simulink model "formation_planner_exp_cs"  (R2022b)
settings: Solver=ode5  StartTime=0.0  StopTime=80  FixedStep=1/1000  RelTol=1e-3
PreLoadFcn:
  | mbxruntime.callbacks.PreLoadFcn(bdroot);
PostLoadFcn:
  | mbxruntime.callbacks.PostLoadFcn(bdroot);
InitFcn:
  | mbxruntime.callbacks.InitFcn(bdroot);
StartFcn:
  | mbxruntime.callbacks.StartFcn(bdroot);
StopFcn:
  | mbxruntime.callbacks.StopFcn(bdroot);
model workspace (MAT data in the model file):
  mbox_table : object (value not decoded)
  model_closed = 0
  sim_status = 0
values from neighbouring files (symbols this model uses):
  c_factor = 43.75    [emplanner_init.m]
  car1_s = -10    [emplanner_init.m]
  car2_s = -20    [emplanner_init.m]
  cf = -175016    [emplanner_init.m]
  cr = -130634    [emplanner_init.m]
  KD_PID_distance = 0.0    (= 0)    [emplanner_init.m]
  KD_PID_speed = 0    [emplanner_init.m]
  KI_PID_distance = 0.0    (= 0)    [emplanner_init.m]
  KI_PID_speed = 0    [emplanner_init.m]
  KP_PID_distance = 0.5    [emplanner_init.m]
  KP_PID_speed = 1.8    [emplanner_init.m]
  la = 1.265    [emplanner_init.m]
  lb = 2.947-1.265    (= 1.682)    [emplanner_init.m]
  leader_global_kappa = global_kappa    [kappa.m]    (also in leader_global_path.mat = [0 0 0 0 0 0 0 0 0 0 0 0 ... (801 elements, 801x1)])
  leader_global_path_x = x_orgin.Data    [kappa.m]    (also in leader_global_path.mat = [2.22044604925e-16 0.999382255067 1.99750536558 2.9943522493)
  leader_global_path_y = y.Data    [kappa.m]    (also in leader_global_path.mat = [2 2 2 2 2 2 2 2 2 2 2 2 ... (801 elements, 801x1)])
  leader_global_yaw = yaw.Data    [kappa.m]    (also in leader_global_path.mat = [0 0 0 0 0 0 0 0 0 0 0 0 ... (801 elements, 801x1)])
  LQR_K1 = k(:,1)'    [emplanner_init.m]
  LQR_K2 = k(:,2)'    [emplanner_init.m]
  LQR_K3 = k(:,3)'    [emplanner_init.m]
  LQR_K4 = k(:,4)'    [emplanner_init.m]
  m = 2020    [emplanner_init.m]
  rack_displacement = [-39.14 , -37.2 , -35.29 , -33.43 , -31.6 , -29.81 , -28.06 , -26.34 , -24.66 ,      -23.01 , -21.38 , -19.79 , -18.23 , -16.69 , -15.18 , -13.7 , -12.23 , -10.8 , -9.38 , -7.98 ,     -6.61 , -5.25 , -3.91 , -2.59 , -1.29 , 0 , 1.27 , 2.54 , 3.78 , 5.02 , 6.24 , 7.46 , 8.66 ,      9.86 , 11.05 , 12.24 , 13.41 , 14.59 , 15.76 , 16.92 , 18.09 , 19.25 , 20.42 , 21.59 , 22.76 ,      23.93 , 25.11 , 26 ...(+26 chars)    [emplanner_init.m]
  right_wheel_ground = [-70 ,-67.2 , -64.4 , -61.6 , -58.8 , -56 , -53.2 , -50.4 , -47.6 , -44.8 , -42 ,      -39.2 , -36.4 , -33.6 , -30.8 , -28 , -25.2 , -22.4 , -19.6 , -16.8 , -14 , -11.2 , -8.4 , -5.6 ,      -2.8 , 0 , 2.8 , 5.6 , 8.4 , 11.2 , 14 , 16.8 , 19.6 , 22.4 , 25.2 , 28 , 30.8 , 33.6 , 36.4 ,      39.2 , 42 , 44.8 , 47.6 , 50.4 , 53.2 , 56 , 58.8 , 61.6 , 64.4 , 67.2 , 70 ]    [emplanner_init.m]
  vx_break_point = zeros(1,5000)    [emplanner_init.m]
undefined symbols (not defined in the file or in its folder): aubr, car1_global_kappa, car1_global_path_x, car1_global_path_y, car1_global_yaw, car2_global_kappa, car2_global_path_x, car2_global_path_y, car2_global_yaw, DiscIntNeverNeededParam, tablebr, vubr, warningInitialVelocity, x0
libraries: PreScanSimulinkLibrary x65, simulink x19, simulink_extras x14, Solver_SF x2
(part 12 of 31)

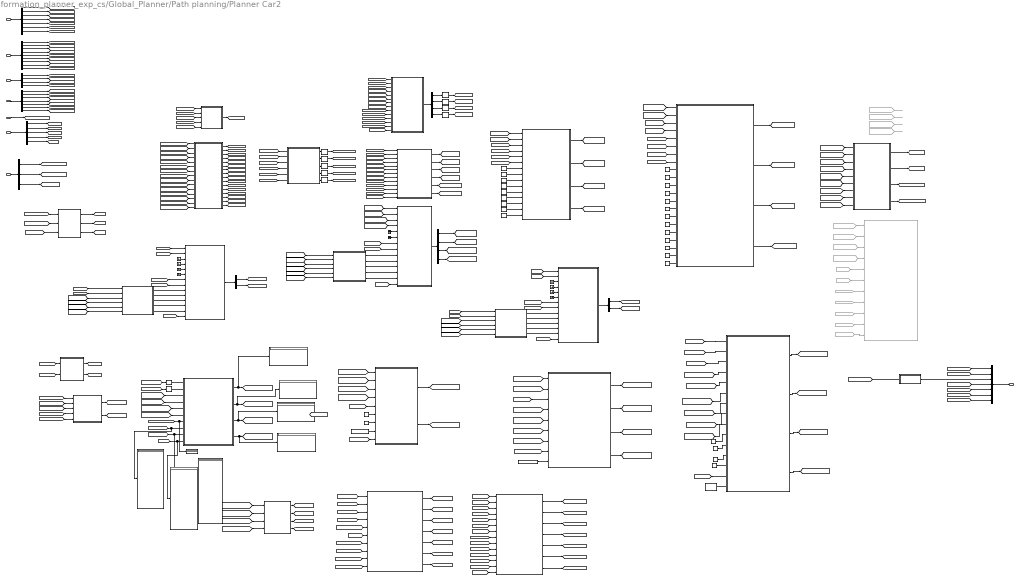
== system formation_planner_exp_cs/Global_Planner/Path planning/Planner Car2 ==
  referenceline info : Inport
  location info : Inport  Port=2
  perception info : Inport  Port=3
  pre_planning info : Inport  Port=4
  current time : Inport  Port=5
  leader_location_info : Inport  Port=6
  pre_car_result : Inport  Port=7
  Bus Creator : BusCreator  Inputs=7
  Bus Selector : BusSelector  OutputSignals=referenceline_x,referenceline_y,referenceline_heading,referenceline_kappa,origin_match_point_index,origin_x,origin_y
  Bus Selector1 : BusSelector  OutputSignals=host_x,host_y,host_heading_xy,host_vx,host_vy,host_yawrate,host_speed,host_ax,host_ay
  Bus Selector2 : BusSelector  OutputSignals=obs_x_set_gcs,obs_y_set_gcs,obs_velocity_set_gcs,obs_heading_set_gcs
  Bus Selector3 : BusSelector  OutputSignals=trajectory_x_gcs,trajectory_y_gcs,trajectory_heading_gcs,trajectory_kappa_gcs,trajectory_speed_gcs,trajectory_accel_gcs,trajectory_time_gcs
  Bus Selector4 : BusSelector  OutputSignals=s_set,l_set,dl_set,ddl_set
  Bus Selector5 : BusSelector  OutputSignals=s_set,l_set,s_dot_set,l_dot_set
  Bus Selector6 : BusSelector  OutputSignals=leader_x,leader_y,end_leader_x,end_leader_y,detla_t
  Bus Selector7 : BusSelector  OutputSignals=s_set,l_set
  Bus Selector8 : BusSelector  OutputSignals=trajectory_x_gcs,trajectory_y_gcs,trajectory_time_gcs
  Bus Selector9 : BusSelector  OutputSignals=s_set,l_set
  Cartesian2Frenet : Subsystem
  Cartesian2Frenet1 : Subsystem
  Cartesian2Frenet2 : Subsystem
  Cartesian2Frenet3 : Subsystem
  Constant : Constant  Value=1e6
  Constant1 : Constant  Value=2000
  Constant10 : Constant  Value=0.1
  Constant11 : Constant  Value=0.02
  Constant12 : Constant  Value=5
  Constant13 : Constant  Value=25000
  Constant14 : Constant  Value=50
  Constant15 : Constant  Value=20
  Constant{7,16..19} (5 alike) : Constant  Value=15
  Constant2 : Constant  Value=2
  Constant20 : Constant  Value=3
  Constant21 : Constant  Value=3
  Constant22 : Constant  Value=1.63
  Constant23 : Constant  Value=10
  Constant24 : Constant  Value=400
  Constant25 : Constant  Value=100
  Constant26 : Constant  Value=1000000000
  Constant27 : Constant  Value=0.2*9.8
  Constant28 : Constant  Value=50
  Constant29 : Constant  Value=500
  Constant3 : Constant  Value=3
  Constant30 : Constant  Value=20
  Constant34 : Constant  Value=car2_s
  Constant4 : Constant  Value=10
  Constant5 : Constant  Value=11
  Constant6 : Constant  Value=4
  Constant8 : Constant
  Constant9 : Constant  Value=10
  Delay : Delay  DelayLength=1
  Delay1 : Delay  DelayLength=1
  Display{,1..7} (8 alike) : Display
  Frenet2Cartesian task : MATLAB Function  TreatAsAtomicUnit=on
  From103 : From  Commented=on  GotoTag=dp_path_s_final
  From109 : From  Commented=on  GotoTag=dp_path_l_final
  From116 : From  Commented=on  GotoTag=dp_path_dl_final
  From117 : From  Commented=on  GotoTag=dp_path_ddl_final
  From120 : From  Commented=on  GotoTag=dp_path_s_final
  From124 : From  Commented=on  GotoTag=dp_path_l_final
  From125 : From  Commented=on  GotoTag=l_min
  From126 : From  Commented=on  GotoTag=l_max
  From129 : From  Commented=on  GotoTag=plan_start_l
  From130 : From  Commented=on  GotoTag=plan_start_dl
  From131 : From  Commented=on  GotoTag=plan_start_s
  From132 : From  Commented=on  GotoTag=static_obs_s_set
  From133 : From  Commented=on  GotoTag=static_obs_l_set
  From91 : From  Commented=on  GotoTag=qp_path_s_final
  From92 : From  Commented=on  GotoTag=qp_path_l_final
  Ground{,1..9} (10 alike) : Ground
  MATLAB Function : MATLAB Function  TreatAsAtomicUnit=on
  MATLAB Function1 : MATLAB Function  TreatAsAtomicUnit=on
  MATLAB Function2 : MATLAB Function  TreatAsAtomicUnit=on
  MATLAB Function3 : MATLAB Function  TreatAsAtomicUnit=on
  MATLAB Function4 : MATLAB Function  TreatAsAtomicUnit=on
  MATLAB Function5 : MATLAB Function  TreatAsAtomicUnit=on
  Selector{1..9} (9 alike) : Selector  InputPortWidth=128  IndexOptions=Index vector (dialog)  Indices=1  OutputSizes=1
  calc path length and map between point and s1 : MATLAB Function  TreatAsAtomicUnit=on
  calc plan start info and stitch trajectory : MATLAB Function  TreatAsAtomicUnit=on
  calc speed planning start condition : MATLAB Function  TreatAsAtomicUnit=on
  generate convex space : MATLAB Function  TreatAsAtomicUnit=on
  generate st graph : MATLAB Function  TreatAsAtomicUnit=on
  genrate index to s : MATLAB Function  TreatAsAtomicUnit=on
  increase st point count : MATLAB Function  TreatAsAtomicUnit=on
  obs : Subsystem
  path and speed merge : MATLAB Function  TreatAsAtomicUnit=on
  path decision task : Subsystem
  path planning task : Subsystem
  plot : MATLAB Function  Commented=on  TreatAsAtomicUnit=on
  speed decision with dynamic planning(dp) : MATLAB Function  TreatAsAtomicUnit=on
  speed planning with quadratic programming (qp) : MATLAB Function  TreatAsAtomicUnit=on
  stitch trajectory : MATLAB Function  TreatAsAtomicUnit=on
  EM Planner result : Outport
  wires:
  Constant30/1 -> speed planning with quadratic programming (qp)/13(w_cost_follow)
  [leader_poj_s] -> speed planning with quadratic programming (qp)/1(leader_poj_s)
  [trajectory_heading_init] -> MATLAB Function3/5(frenet_path_heading)
  MATLAB Function3/3(proj_y_set) -> Cartesian2Frenet2/11(proj_y_set)
  [trajectory_x_init] -> MATLAB Function3/3(frenet_path_x)
  MATLAB Function3/1(match_point_index_set) -> Cartesian2Frenet2/9(proj_match_point_index_set)
  MATLAB Function3/2(proj_x_set) -> Cartesian2Frenet2/10(proj_x_set)
  [trajectory_kappa_init] -> MATLAB Function3/6(frenet_path_kappa)
  [trajectory_x_init] -> Cartesian2Frenet2/7(frenet_path_x)
  [trajectory_y_init] -> Cartesian2Frenet2/8(frenet_path_y)
  [leader_start_x] -> MATLAB Function3/1(x_set)
  [leader_start_y] -> MATLAB Function3/2(y_set)
  MATLAB Function3/4(proj_heading_set) -> Cartesian2Frenet2/12(proj_heading_set)
  MATLAB Function3/5(proj_kappa_set) -> Cartesian2Frenet2/13(proj_kappa_set)
  [trajectory_y_init] -> MATLAB Function3/4(frenet_path_y)
  Bus Selector7/1 -> [leader_poj_s]  "<s_set>"
  [leader_start_x] -> Cartesian2Frenet2/1(x_set)
  Ground3/1 -> Cartesian2Frenet2/4(vy_set)
  Ground4/1 -> Cartesian2Frenet2/5(ax_set)
  Cartesian2Frenet2/1(Cartesian2FrenetOut) -> Bus Selector7/1
  Bus Selector7/2 -> [leader_poj_l]  "<l_set>"
  Ground5/1 -> Cartesian2Frenet2/6(ay_set)
  [leader_start_y] -> Cartesian2Frenet2/2(y_set)
  [path_index2s] -> Cartesian2Frenet2/14(index2s)
  Ground2/1 -> Cartesian2Frenet2/3(vx_set)
  Bus Selector6/5 -> [detla_t]  "<detla_t>"
  Bus Selector6/4 -> [leader_end_y]  "<end_leader_y>"
  Bus Selector6/3 -> [leader_end_x]  "<end_leader_x>"
  Bus Selector6/2 -> [leader_start_y]  "<leader_y>"
  Bus Selector6/1 -> [leader_start_x]  "<leader_x>"
  leader_location_info/1 -> Bus Selector6/1
  [host_speed] -> obs/4(host_speed)
  From109/1 -> ?
  From116/1 -> ?
  From117/1 -> ?
  From103/1 -> ?
  [qp_path_dl_final] -> Frenet2Cartesian task/3(dl_set)
  [qp_path_s_final] -> Frenet2Cartesian task/1(s_set)
  [qp_path_l_final] -> Frenet2Cartesian task/2(l_set)
  [qp_path_ddl_final] -> Frenet2Cartesian task/4(ddl_set)
  stitch trajectory/6(trajectory_accel_final) -> [trajectory_accel_final]
  [s_dot_lb] -> speed planning with quadratic programming (qp)/8(s_dot_lb)
  generate convex space/3(s_dot_lb) -> [s_dot_lb]
  generate st graph/1(obs_st_s_in_set) -> Display/1, [obs_st_s_in_set]
  [s] -> Delay/1
  [dp_speed_s] -> speed planning with quadratic programming (qp)/4(dp_speed_s)
  Constant29/1 -> speed planning with quadratic programming (qp)/12(w_cost_jerk)
  [stitch_y_gcs] -> stitch trajectory/9(stitch_y)
  Constant25/1 -> speed decision with dynamic planning(dp)/7(w_cost_accel)
  speed decision with dynamic planning(dp)/1(dp_speed_s) -> [dp_speed_s]
  [obs_st_t_out_set] -> speed decision with dynamic planning(dp)/4(obs_st_t_out_set)
  Constant23/1 -> [reference_speed]
  [dp_speed_t] -> speed planning with quadratic programming (qp)/5(dp_speed_t)
  [trajectory_heading] -> stitch trajectory/3(trajectory_heading)
  [plan_start_ay_gcs] -> calc speed planning start condition/4(plan_start_ay)
  [relative_time_init] -> increase st point count/4(relative_time_init)
  path and speed merge/1(trajectory_x) -> [trajectory_x]
  [trajectory_accel] -> stitch trajectory/6(trajectory_accel)
  [plan_start_ax_gcs] -> calc speed planning start condition/3(plan_start_ax)
  [stitch_speed_gcs] -> stitch trajectory/12(stitch_speed)
  [trajectory_speed] -> stitch trajectory/5(trajectory_speed)
  stitch trajectory/4(trajectory_kappa_final) -> [trajectory_kappa_final]
  speed planning with quadratic programming (qp)/4(relative_time_init) -> [relative_time_init]
  speed planning with quadratic programming (qp)/2(qp_s_dot_init) -> [qp_s_dot_init]
  [reference_speed] -> speed decision with dynamic planning(dp)/5(reference_speed_unlimit)
  [plan_start_s_dot] -> speed planning with quadratic programming (qp)/2(plan_start_s_dot)
  stitch trajectory/1(trajectory_x_final) -> [trajectory_x_final]
  [stitch_heading_gcs] -> stitch trajectory/10(stitch_heading)
  [stitch_accel_gcs] -> stitch trajectory/13(stitch_accel)
  [stitch_kappa_gcs] -> stitch trajectory/11(stitch_kappa)
  [stitch_time] -> stitch trajectory/14(stitch_time)
  [qp_s_init] -> increase st point count/1(s_init)
  [obs_st_s_in_set] -> speed decision with dynamic planning(dp)/1(obs_st_s_in_set)
  generate convex space/4(s_dot_ub) -> [s_dot_ub]
  [trajectory_y] -> stitch trajectory/2(trajectory_y)
  path and speed merge/2(trajectory_y) -> [trajectory_y]
  generate convex space/1(s_lb) -> [s_lb]
  [trajectory_kappa_init] -> path and speed merge/10(trajectory_kappa_init)
  path and speed merge/3(trajectory_heading) -> [trajectory_heading]
  [plan_start_s_dot2] -> speed planning with quadratic programming (qp)/3(plan_start_s_dot2)
  [trajectory_kappa] -> stitch trajectory/4(trajectory_kappa)
  [obs_st_s_in_set] -> generate convex space/4(obs_st_s_in_set)
  [trajectory_time] -> stitch trajectory/7(trajectory_time)
  [plan_start_time] -> path and speed merge/5(current_time)
  [s_ub] -> speed planning with quadratic programming (qp)/7(s_ub)
  [trajectory_y_init] -> path and speed merge/8(trajectory_y_init)
  [s_lb] -> speed planning with quadratic programming (qp)/6(s_lb)
  [trajectory_heading_init] -> path and speed merge/9(trajectory_heading_init)
  [path_index2s] -> path and speed merge/6(path_s)
  [qp_s_dot2_init] -> increase st point count/3(s_dot2_init)
  path and speed merge/5(trajectory_speed) -> [trajectory_speed]
  path and speed merge/7(trajectory_time) -> [trajectory_time]
  Constant26/1 -> speed decision with dynamic planning(dp)/8(w_cost_obs)
  [plan_start_heading_gcs] -> calc speed planning start condition/5(plan_start_heading)
  [obs_st_s_out_set] -> speed decision with dynamic planning(dp)/2(obs_st_s_out_set)
  Constant27/1 -> generate convex space/9(max_lateral_accel)
  [stitch_x_gcs] -> stitch trajectory/8(stitch_x)
  generate st graph/2(obs_st_s_out_set) -> Display1/1, [obs_st_s_out_set]
  speed decision with dynamic planning(dp)/2(dp_speed_t) -> [dp_speed_t]
  Constant9/1 -> speed planning with quadratic programming (qp)/10(w_cost_s_dot2)
  generate st graph/3(obs_st_t_in_set) -> Display2/1, [obs_st_t_in_set]
  speed planning with quadratic programming (qp)/1(qp_s_init) -> [qp_s_init]
  [relative_time] -> Delay1/1
  stitch trajectory/2(trajectory_y_final) -> [trajectory_y_final]
  [dynamic_obs_l_dot_set] -> generate st graph/6(dynamic_obs_l_dot_set)
  [s_dot_ub] -> speed planning with quadratic programming (qp)/9(s_dot_ub)
  [obs_st_t_in_set] -> speed decision with dynamic planning(dp)/3(obs_st_t_in_set)
  Constant28/1 -> speed planning with quadratic programming (qp)/11(w_cost_v_ref)
  calc speed planning start condition/1(plan_start_s_dot) -> [plan_start_s_dot]
  [reference_speed] -> speed planning with quadratic programming (qp)/14(speed_reference)
  speed planning with quadratic programming (qp)/3(qp_s_dot2_init) -> [qp_s_dot2_init]
  path and speed merge/4(trajectory_kappa) -> [trajectory_kappa]
  [dynamic_obs_s_dot_set] -> generate st graph/5(dynamic_obs_s_dot_set)
  [qp_s_dot_init] -> increase st point count/2(s_dot_init)
  [plan_start_s_dot] -> speed decision with dynamic planning(dp)/9(plan_start_s_dot)
  generate convex space/2(s_ub) -> [s_ub]
  [trajectory_kappa_init] -> generate convex space/8(trajectory_kappa_init)
  [obs_st_s_out_set] -> generate convex space/5(obs_st_s_out_set)
  [obs_st_t_out_set] -> generate convex space/7(obs_st_t_out_set)
  [obs_st_t_in_set] -> generate convex space/6(obs_st_t_in_set)
  [plan_start_vx_gcs] -> calc speed planning start condition/1(plan_start_vx)
  stitch trajectory/3(trajectory_heading_final) -> [trajectory_heading_final]
  [plan_start_vy_gcs] -> calc speed planning start condition/2(plan_start_vy)
  [s] -> path and speed merge/1(s)
  increase st point count/1(s) -> [s]
  [s_dot] -> path and speed merge/2(s_dot)
  [s_dot2] -> path and speed merge/3(s_dot2)
  [trajectory_x_init] -> path and speed merge/7(trajectory_x_init)
  calc speed planning start condition/2(plan_start_s_dot2) -> [plan_start_s_dot2]
  [relative_time] -> path and speed merge/4(relative_time)
  [trajectory_x] -> stitch trajectory/1(trajectory_x)
  path and speed merge/6(trajectory_accel) -> [trajectory_accel]
  Constant24/1 -> speed decision with dynamic planning(dp)/6(w_cost_ref_speed)
  generate st graph/4(obs_st_t_out_set) -> Display3/1, [obs_st_t_out_set]
  Delay1/1 -> generate st graph/2(pre_trajectory_t)
  stitch trajectory/7(trajectory_time_final) -> [trajectory_time_final]
  Delay/1 -> generate st graph/1(pre_trajectory_s)
  [dynamic_obs_s_set] -> generate st graph/3(dynamic_obs_s_set)
  increase st point count/3(s_dot2) -> [s_dot2]
  [path_index2s] -> generate convex space/3(path_index2s)
  stitch trajectory/5(trajectory_speed_final) -> [trajectory_speed_final]
  increase st point count/2(s_dot) -> [s_dot]
  [dynamic_obs_l_set] -> generate st graph/4(dynamic_obs_l_set)
  [dp_speed_s] -> generate convex space/1(dp_speed_s)
  increase st point count/4(relative_time) -> [relative_time]
  [dp_speed_t] -> generate convex space/2(dp_speed_t)
  Bus Selector5/4 -> [dynamic_obs_l_dot_set]  "<l_dot_set>"
  [dynamic_obs_x_set] -> Cartesian2Frenet1/1(x_set)
  Bus Selector5/3 -> [dynamic_obs_s_dot_set]  "<s_dot_set>"
  [trajectory_heading_init] -> MATLAB Function1/5(frenet_path_heading)
  [dynamic_obs_y_set] -> MATLAB Function1/2(y_set)
  [trajectory_y_init] -> Cartesian2Frenet1/8(frenet_path_y)
  Bus Selector5/2 -> [dynamic_obs_l_set]  "<l_set>"
  MATLAB Function1/1(match_point_index_set) -> Cartesian2Frenet1/9(proj_match_point_index_set)
  [trajectory_kappa_init] -> MATLAB Function1/6(frenet_path_kappa)
  Ground/1 -> Cartesian2Frenet1/5(ax_set)
  [path_index2s] -> Cartesian2Frenet1/14(index2s)
  [trajectory_x_init] -> Cartesian2Frenet1/7(frenet_path_x)
  Cartesian2Frenet1/1(Cartesian2FrenetOut) -> Bus Selector5/1
  MATLAB Function1/3(proj_y_set) -> Cartesian2Frenet1/11(proj_y_set)
  [dynamic_obs_vy_set] -> Cartesian2Frenet1/4(vy_set)
  [dynamic_obs_y_set] -> Cartesian2Frenet1/2(y_set)
  [dynamic_obs_vx_set] -> Cartesian2Frenet1/3(vx_set)
  [trajectory_y_init] -> MATLAB Function1/4(frenet_path_y)
  MATLAB Function1/2(proj_x_set) -> Cartesian2Frenet1/10(proj_x_set)
  MATLAB Function1/4(proj_heading_set) -> Cartesian2Frenet1/12(proj_heading_set)
  Ground1/1 -> Cartesian2Frenet1/6(ay_set)
  [dynamic_obs_x_set] -> MATLAB Function1/1(x_set)
  MATLAB Function1/5(proj_kappa_set) -> Cartesian2Frenet1/13(proj_kappa_set)
  [trajectory_x_init] -> MATLAB Function1/3(frenet_path_x)
  Bus Selector5/1 -> [dynamic_obs_s_set]  "<s_set>"
  calc path length and map between point and s1/1(path_s_end) -> [path_s_end]
  [trajectory_y_init] -> calc path length and map between point and s1/2(trajectory_y)
  calc path length and map between point and s1/2(path_index2s) -> [path_index2s]
  [trajectory_x_init] -> calc path length and map between point and s1/1(trajectory_x)
  [obs_x_set_gcs] -> obs/5(obs_x_set_gcs)
  obs/1(static_obs_s_set) -> [static_obs_s_set]
  [obs_y_set_gcs] -> obs/6(obs_y_set_gcs)
  [host_x] -> obs/1(host_x)
  [host_y] -> obs/2(host_y)
  [referenceline_kappa] -> obs/12(referenceline_kappa)
  [referenceline_heading] -> obs/11(referenceline_heading)
  [referenceline_x] -> obs/9(referenceline_x)
  [obs_heading_set_gcs] -> obs/8(obs_heading_set_gcs)
  [host_heading_xy] -> obs/3(host_heading_xy)
  [referenceline_y] -> obs/10(referenceline_y)
  [index2s] -> obs/13(index2s)
  obs/2(static_obs_l_set) -> [static_obs_l_set]
  obs/4(dynamic_obs_y_set) -> [dynamic_obs_y_set]
  obs/5(dynamic_obs_vx_set) -> [dynamic_obs_vx_set]
  obs/3(dynamic_obs_x_set) -> [dynamic_obs_x_set]
  obs/6(dynamic_obs_vy_set) -> [dynamic_obs_vy_set]
  [obs_velocity_set_gcs] -> obs/7(obs_velocity_set_gcs)
  MATLAB Function/1(y) -> Bus Creator/3  "trajectory_heading_gcs"
  [plan_start_s] -> path planning task/5(plan_start_s)
  From92/1 -> plot/4(qp_l)
  From91/1 -> plot/3(qp_s)
  path planning task/4(qp_path_ddl_final) -> [qp_path_ddl_final]
  path planning task/3(qp_path_dl_final) -> [qp_path_dl_final]
  path planning task/2(qp_path_l_final) -> [qp_path_l_final]
  path planning task/1(qp_path_s_final) -> [qp_path_s_final]
  Constant11/1 -> path planning task/21(delta_ddl_max)
  Constant10/1 -> path planning task/20(delta_dl_max)
  [static_obs_l_set] -> path planning task/4(static_obs_l_set)
  [static_obs_s_set] -> path planning task/3(static_obs_s_set)
  Constant2/1 -> path decision task/9(dp_cost_ddl)
  Constant1/1 -> path decision task/8(dp_cost_dl)
  Constant/1 -> path decision task/7(dp_cost_collision)
  Constant3/1 -> path decision task/10(dp_cost_dddl)
  Constant4/1 -> path decision task/11(dp_cost_ref)
  Constant5/1 -> path decision task/12(dp_row)
  Constant6/1 -> path decision task/13(dp_col)
  Constant7/1 -> path decision task/14(dp_sample_s)
  Constant8/1 -> path decision task/15(dp_sample_l)
  Constant12/1 -> path planning task/9(qp_cost_l)
  Constant13/1 -> path planning task/10(qp_cost_dl)
  Constant14/1 -> path planning task/11(qp_cost_ddl)
  Constant15/1 -> path planning task/12(qp_cost_dddl)
  Constant16/1 -> path planning task/13(qp_cost_centre)
  Constant17/1 -> path planning task/14(qp_cost_endl)
  Constant18/1 -> path planning task/15(qp_cost_end_dl)
  Constant19/1 -> path planning task/16(qp_cost_end_ddl)
  Constant20/1 -> path planning task/17(host_d1)
  Constant21/1 -> path planning task/18(host_d2)
  Constant22/1 -> path planning task/19(host_w)
  [plan_start_dl] -> path planning task/7(plan_start_dl)
  [plan_start_ddl] -> path planning task/8(plan_start_ddl)
  [plan_start_l] -> path planning task/6(plan_start_l)
  [dp_path_l_final] -> path planning task/2(dp_path_l_final)
  [dp_path_s_final] -> path planning task/1(dp_path_s_final)
  [plan_start_s] -> path decision task/3(plan_start_s)
  [plan_start_l] -> path decision task/4(plan_start_l)
  [plan_start_dl] -> path decision task/5(plan_start_dl)
  [plan_start_ddl] -> path decision task/6(plan_start_ddl)
  [static_obs_l_set] -> path decision task/2(static_obs_l_set)
  [static_obs_s_set] -> path decision task/1(static_obs_s_set)
  path decision task/4(dp_path_ddl_final) -> [dp_path_ddl_final]
  path decision task/3(dp_path_dl_final) -> [dp_path_dl_final]
  path decision task/2(dp_path_l_final) -> [dp_path_l_final]
  path decision task/1(dp_path_s_final) -> [dp_path_s_final]
  From133/1 -> plot/8(obs_l_set)
  From132/1 -> plot/7(obs_s_set)
  From131/1 -> plot/9(start_s)
  From129/1 -> plot/10(start_l)
  From130/1 -> plot/11(start_dl)
  From126/1 -> plot/6(l_max)
  From125/1 -> plot/5(l_min)
  From124/1 -> plot/2(dp_l)
  From120/1 -> plot/1(dp_s)
  Frenet2Cartesian task/4(kappa_set) -> [trajectory_kappa_init]
  Frenet2Cartesian task/3(heading_set) -> [trajectory_heading_init]
  Frenet2Cartesian task/2(y_set) -> [trajectory_y_init]
  Frenet2Cartesian task/1(x_set) -> [trajectory_x_init]
  [referenceline_kappa] -> Frenet2Cartesian task/8(frenet_path_kappa)
  [referenceline_heading] -> Frenet2Cartesian task/7(frenet_path_heading)
  [referenceline_y] -> Frenet2Cartesian task/6(frenet_path_y)
  [referenceline_x] -> Frenet2Cartesian task/5(frenet_path_x)
  [index2s] -> Frenet2Cartesian task/9(index2s)
  [trajectory_y_final] -> Bus Creator/2  "trajectory_y_gcs"
  [trajectory_kappa_final] -> Bus Creator/4  "trajectory_kappa_gcs"
  [trajectory_heading_final] -> MATLAB Function/1(trajectory_heading_final)
  [trajectory_speed_final] -> Bus Creator/5  "trajectory_speed_gcs"
  [trajectory_accel_final] -> Bus Creator/6  "trajectory_accel_gcs"
  [trajectory_time_final] -> Bus Creator/7  "trajectory_time_gcs"
  [trajectory_x_final] -> Bus Creator/1  "trajectory_x_gcs"
  Bus Creator/1 -> EM Planner result/1
  [index2s] -> Cartesian2Frenet/14(index2s)
  Selector9/1 -> [plan_start_ddl]
  Selector8/1 -> [plan_start_dl]
  Selector7/1 -> [plan_start_l]
  Selector6/1 -> [plan_start_s]
  Bus Selector4/1 -> Selector6/1  "<s_set>"
  Bus Selector4/2 -> Selector7/1  "<l_set>"
  Bus Selector4/3 -> Selector8/1  "<dl_set>"
  Bus Selector4/4 -> Selector9/1  "<ddl_set>"
  Cartesian2Frenet/1(Cartesian2FrenetOut) -> Bus Selector4/1
  [plan_start_proj_kappa] -> Cartesian2Frenet/13(proj_kappa_set)
  [plan_start_proj_heading] -> Cartesian2Frenet/12(proj_heading_set)
  [plan_start_proj_y] -> Cartesian2Frenet/11(proj_y_set)
  [plan_start_proj_x] -> Cartesian2Frenet/10(proj_x_set)
  [plan_start_match_point_index] -> Cartesian2Frenet/9(proj_match_point_index_set)
  [referenceline_y] -> Cartesian2Frenet/8(frenet_path_y)
  [referenceline_x] -> Cartesian2Frenet/7(frenet_path_x)
  [plan_start_ay_gcs] -> Cartesian2Frenet/6(ay_set)
  [plan_start_ax_gcs] -> Cartesian2Frenet/5(ax_set)
  [plan_start_vy_gcs] -> Cartesian2Frenet/4(vy_set)
  [plan_start_vx_gcs] -> Cartesian2Frenet/3(vx_set)
  [plan_start_x_gcs] -> Cartesian2Frenet/1(x_set)
  [plan_start_y_gcs] -> Cartesian2Frenet/2(y_set)
  Selector5/1 -> [plan_start_proj_kappa]
  Selector4/1 -> [plan_start_proj_heading]
  Selector3/1 -> [plan_start_proj_y]
  Selector2/1 -> [plan_start_proj_x]
  Selector1/1 -> [plan_start_match_point_index]
  [referenceline_kappa] -> MATLAB Function2/6(frenet_path_kappa)
  [referenceline_heading] -> MATLAB Function2/5(frenet_path_heading)
  [referenceline_y] -> MATLAB Function2/4(frenet_path_y)
  [referenceline_x] -> MATLAB Function2/3(frenet_path_x)
  [plan_start_y_gcs] -> MATLAB Function2/2(y_set)
  [plan_start_x_gcs] -> MATLAB Function2/1(x_set)
  MATLAB Function2/2(proj_x_set) -> Selector2/1
  MATLAB Function2/4(proj_heading_set) -> Selector4/1
  MATLAB Function2/1(match_point_index_set) -> Selector1/1
  MATLAB Function2/3(proj_y_set) -> Selector3/1
  MATLAB Function2/5(proj_kappa_set) -> Selector5/1
  genrate index to s/1(index2s) -> [index2s]
  [origin_match_point_index] -> genrate index to s/5(origin_match_point_index)
  [origin_y] -> genrate index to s/4(origin_y)
  [origin_x] -> genrate index to s/3(origin_x)
  [referenceline_y] -> genrate index to s/2(path_y)
  [referenceline_x] -> genrate index to s/1(path_x)
  Bus Selector/7 -> [origin_y]  "<origin_y>"
  Bus Selector/6 -> [origin_x]  "<origin_x>"
  Bus Selector/5 -> [origin_match_point_index]  "<origin_match_point_index>"
  calc plan start info and stitch trajectory/16(stitch_time) -> [stitch_time]
  calc plan start info and stitch trajectory/15(stitch_accel) -> [stitch_accel_gcs]
  calc plan start info and stitch trajectory/14(stitch_speed) -> [stitch_speed_gcs]
  calc plan start info and stitch trajectory/13(stitch_kappa) -> [stitch_kappa_gcs]
  calc plan start info and stitch trajectory/12(stitch_heading) -> [stitch_heading_gcs]
  calc plan start info and stitch trajectory/11(stitch_y) -> [stitch_y_gcs]
  calc plan start info and stitch trajectory/10(stitch_x) -> [stitch_x_gcs]
  calc plan start info and stitch trajectory/9(plan_start_time) -> [plan_start_time]
  calc plan start info and stitch trajectory/8(plan_start_ay) -> [plan_start_ay_gcs]
  calc plan start info and stitch trajectory/7(plan_start_ax) -> [plan_start_ax_gcs]
  calc plan start info and stitch trajectory/6(plan_start_vy) -> [plan_start_vy_gcs]
  calc plan start info and stitch trajectory/5(plan_start_vx) -> [plan_start_vx_gcs]
  calc plan start info and stitch trajectory/4(plan_start_kappa) -> [plan_start_kappa_gcs]
  calc plan start info and stitch trajectory/3(plan_start_heading) -> [plan_start_heading_gcs]
  calc plan start info and stitch trajectory/2(plan_start_y) -> [plan_start_y_gcs]
  calc plan start info and stitch trajectory/1(plan_start_x) -> [plan_start_x_gcs]
  [pre_trajectory_heading_gcs] -> calc plan start info and stitch trajectory/3(pre_trajectory_heading)
  [pre_trajectory_kappa_gcs] -> calc plan start info and stitch trajectory/4(pre_trajectory_kappa)
  [pre_trajectory_speed_gcs] -> calc plan start info and stitch trajectory/5(pre_trajectory_velocity)
  [pre_trajectory_accel_gcs] -> calc plan start info and stitch trajectory/6(pre_trajectory_accel)
  [pre_trajectory_time] -> calc plan start info and stitch trajectory/7(pre_trajectory_time)
  [pre_trajectory_y_gcs] -> calc plan start info and stitch trajectory/2(pre_trajectory_y)
  [pre_trajectory_x_gcs] -> calc plan start info and stitch trajectory/1(pre_trajectory_x)
  [current_time] -> calc plan start info and stitch trajectory/8(current_time)
  [host_x] -> calc plan start info and stitch trajectory/9(host_x)
  [host_y] -> calc plan start info and stitch trajectory/10(host_y)
  [host_heading_xy] -> calc plan start info and stitch trajectory/11(host_heading_xy)
  [host_vx_vcs] -> calc plan start info and stitch trajectory/12(host_vx)
  [host_vy_vcs] -> calc plan start info and stitch trajectory/13(host_vy)
  [host_ax_vcs] -> calc plan start info and stitch trajectory/14(host_ax)
  [host_ay_vcs] -> calc plan start info and stitch trajectory/15(host_ay)
  Bus Selector/4 -> [referenceline_kappa]  "<referenceline_kappa>"
  Bus Selector/3 -> [referenceline_heading]  "<referenceline_heading>"
  Bus Selector/2 -> [referenceline_y]  "<referenceline_y>"
  Bus Selector/1 -> [referenceline_x]  "<referenceline_x>"
  Bus Selector1/9 -> [host_ay_vcs]  "<host_ay>"
  Bus Selector1/8 -> [host_ax_vcs]  "<host_ax>"
  Bus Selector1/7 -> [host_speed]  "<host_speed>"
  Bus Selector1/6 -> [host_yawrate]  "<host_yawrate>"
  Bus Selector1/5 -> [host_vy_vcs]  "<host_vy>"
  Bus Selector1/4 -> [host_vx_vcs]  "<host_vx>"
  Bus Selector1/3 -> [host_heading_xy]  "<host_heading_xy>"
  Bus Selector1/2 -> [host_y]  "<host_y>"
  Bus Selector1/1 -> [host_x]  "<host_x>"
  Bus Selector2/4 -> [obs_heading_set_gcs]  "<obs_heading_set_gcs>"
  Bus Selector2/3 -> [obs_velocity_set_gcs]  "<obs_velocity_set_gcs>"
  Bus Selector2/2 -> [obs_y_set_gcs]  "<obs_y_set_gcs>"
  Bus Selector2/1 -> [obs_x_set_gcs]  "<obs_x_set_gcs>"
  Bus Selector3/7 -> [pre_trajectory_time]  "<trajectory_time_gcs>"
  Bus Selector3/6 -> [pre_trajectory_accel_gcs]  "<trajectory_accel_gcs>"
  Bus Selector3/5 -> [pre_trajectory_speed_gcs]  "<trajectory_speed_gcs>"
  Bus Selector3/4 -> [pre_trajectory_kappa_gcs]  "<trajectory_kappa_gcs>"
  Bus Selector3/3 -> [pre_trajectory_heading_gcs]  "<trajectory_heading_gcs>"
  Bus Selector3/2 -> [pre_trajectory_y_gcs]  "<trajectory_y_gcs>"
  Bus Selector3/1 -> [pre_trajectory_x_gcs]  "<trajectory_x_gcs>"
  current time/1 -> [current_time]
  pre_planning info/1 -> Bus Selector3/1
  perception info/1 -> Bus Selector2/1
  location info/1 -> Bus Selector1/1
  referenceline info/1 -> Bus Selector/1
  Constant34/1 -> speed planning with quadratic programming (qp)/15(car_ds)
  Bus Selector8/3 -> [trajecotory_time_pre_car]  "<trajectory_time_gcs>"
  Bus Selector8/2 -> [trajecotory_y_pre_car]  "<trajectory_y_gcs>"
  pre_car_result/1 -> Bus Selector8/1
  Bus Selector8/1 -> [trajecotory_x_pre_car]  "<trajectory_x_gcs>"
  Ground7/1 -> Cartesian2Frenet3/4(vy_set)
  [trajectory_x_init] -> Cartesian2Frenet3/7(frenet_path_x)
  Bus Selector9/2 -> [pre_car_l]  "<l_set>"
  [pre_car_y] -> MATLAB Function4/2(y_set)
  [trajectory_y_init] -> MATLAB Function4/4(frenet_path_y)
  [trajectory_y_init] -> Cartesian2Frenet3/8(frenet_path_y)
  [path_index2s] -> Cartesian2Frenet3/14(index2s)
  MATLAB Function4/5(proj_kappa_set) -> Cartesian2Frenet3/13(proj_kappa_set)
  Ground6/1 -> Cartesian2Frenet3/3(vx_set)
  Ground8/1 -> Cartesian2Frenet3/5(ax_set)
  [trajectory_kappa_init] -> MATLAB Function4/6(frenet_path_kappa)
  Cartesian2Frenet3/1(Cartesian2FrenetOut) -> Bus Selector9/1
  [trajectory_x_init] -> MATLAB Function4/3(frenet_path_x)
  MATLAB Function4/3(proj_y_set) -> Cartesian2Frenet3/11(proj_y_set)
  MATLAB Function4/2(proj_x_set) -> Cartesian2Frenet3/10(proj_x_set)
  [pre_car_y] -> Cartesian2Frenet3/2(y_set)
  [trajectory_heading_init] -> MATLAB Function4/5(frenet_path_heading)
  [pre_car_x] -> Cartesian2Frenet3/1(x_set)
  Bus Selector9/1 -> [pre_car_s]  "<s_set>"
  MATLAB Function4/1(match_point_index_set) -> Cartesian2Frenet3/9(proj_match_point_index_set)
  [pre_car_x] -> MATLAB Function4/1(x_set)
  Ground9/1 -> Cartesian2Frenet3/6(ay_set)
  MATLAB Function4/4(proj_heading_set) -> Cartesian2Frenet3/12(proj_heading_set)
  [pre_car_s] -> Display6/1, generate st graph/8(pre_car_s)
  [pre_car_l] -> Display4/1, generate st graph/9(pre_car_l)
  [current_time] -> Display5/1, generate st graph/7(current_time)
  [pre_car_time] -> Display7/1, generate st graph/10(pre_car_time)
  [trajecotory_x_pre_car] -> MATLAB Function5/1(pre_car_x_init)
  [trajecotory_y_pre_car] -> MATLAB Function5/2(pre_car_y_init)
  [trajecotory_time_pre_car] -> MATLAB Function5/3(pre_car_time_init)
  MATLAB Function5/2(pre_car_y) -> [pre_car_y]
  MATLAB Function5/1(pre_car_x) -> [pre_car_x]
  MATLAB Function5/3(pre_car_time) -> [pre_car_time]

== system formation_planner_exp_cs/Global_Planner/Path planning/car1 referenceline provider ==
  location info : Inport
  Bus Creator : BusCreator  Inputs=7
  Bus Selector : BusSelector  OutputSignals=host_x,host_y,host_heading_xy,host_vx,host_vy,host_yawrate,host_speed
  Constant : Constant  Value=car1_global_path_x
  Constant1 : Constant  Value=car1_global_path_y
  Constant2 : Constant  Value=car1_global_yaw
  Constant3 : Constant  Value=car1_global_kappa
  MATLAB Function2 : MATLAB Function  TreatAsAtomicUnit=on
  MATLAB Function6 : MATLAB Function  TreatAsAtomicUnit=on
  Selector : Selector  InputPortWidth=128  IndexOptions=Index vector (dialog)  Indices=1  OutputSizes=1
  Selector2 : Selector  InputPortWidth=128  IndexOptions=Index vector (dialog)  Indices=1  OutputSizes=1
  Selector3 : Selector  InputPortWidth=128  IndexOptions=Index vector (dialog)  Indices=1  OutputSizes=1
  Terminator_3 : Terminator
  Terminator_4 : Terminator
  referenceline info : Outport
  wires:
  [global_path_x] -> MATLAB Function2/2(global_path_x)
  [host_x] -> MATLAB Function6/1(x_set)
  [global_kappa] -> MATLAB Function6/6(frenet_path_kappa)
  [global_yaw] -> MATLAB Function6/5(frenet_path_heading)
  [global_path_y] -> MATLAB Function6/4(frenet_path_y)
  [global_path_x] -> MATLAB Function6/3(frenet_path_x)
  [host_y] -> MATLAB Function6/2(y_set)
  Selector/1 -> [origin_match_point_index], MATLAB Function2/1(host_match_point_index)
  MATLAB Function6/1(match_point_index_set) -> Selector/1
  [global_path_y] -> MATLAB Function2/3(global_path_y)
  Bus Selector/5 -> [host_vy]  "<host_vy>"
  Bus Selector/1 -> [host_x]  "<host_x>"
  Bus Selector/2 -> [host_y]  "<host_y>"
  Bus Selector/3 -> [host_heading_xy]  "<host_heading_xy>"
  Bus Selector/4 -> [host_vx]  "<host_vx>"
  Bus Selector/7 -> [host_speed]  "<host_speed>"
  Bus Selector/6 -> [host_yawrate]  "<host_yawrate>"
  location info/1 -> Bus Selector/1
  [referenceline_x] -> Bus Creator/1  "referenceline_x"
  [referenceline_y] -> Bus Creator/2  "referenceline_y"
  Bus Creator/1 -> referenceline info/1  "referenceline info"
  [referenceline_kappa] -> Bus Creator/4  "referenceline_kappa"
  [referenceline_heading] -> Bus Creator/3  "referenceline_heading"
  [reference_match_point_index] -> Bus Creator/5  "origin_match_point_index"
  [origin_x] -> Bus Creator/6  "origin_x"
  [origin_y] -> Bus Creator/7  "origin_y"
  MATLAB Function6/4(proj_heading_set) -> Terminator_3/1
  MATLAB Function6/5(proj_kappa_set) -> Terminator_4/1
  Constant/1 -> [global_path_x]
  Constant1/1 -> [global_path_y]
  Constant2/1 -> [global_yaw]
  Constant3/1 -> [global_kappa]
  [global_yaw] -> MATLAB Function2/4(global_heading)
  [global_kappa] -> MATLAB Function2/5(global_kappa)
  MATLAB Function2/1(referenceline_x) -> [referenceline_x]
  MATLAB Function2/2(referenceline_y) -> [referenceline_y]
  MATLAB Function2/3(referenceline_heading) -> [referenceline_heading]
  MATLAB Function2/4(referenceline_kappa) -> [referenceline_kappa]
  Selector3/1 -> [origin_y]
  MATLAB Function6/3(proj_y_set) -> Selector3/1
  MATLAB Function6/2(proj_x_set) -> Selector2/1
  Selector2/1 -> [origin_x]
  MATLAB Function2/5(reference_match_point_index) -> [reference_match_point_index]

== system formation_planner_exp_cs/Global_Planner/Path planning/car2 referenceline provider ==
  location info : Inport
  Bus Creator : BusCreator  Inputs=7
  Bus Selector : BusSelector  OutputSignals=host_x,host_y,host_heading_xy,host_vx,host_vy,host_yawrate,host_speed
  Constant : Constant  Value=car2_global_path_x
  Constant1 : Constant  Value=car2_global_path_y
  Constant2 : Constant  Value=car2_global_yaw
  Constant3 : Constant  Value=car2_global_kappa
  MATLAB Function2 : MATLAB Function  TreatAsAtomicUnit=on
  MATLAB Function6 : MATLAB Function  TreatAsAtomicUnit=on
  Selector : Selector  InputPortWidth=128  IndexOptions=Index vector (dialog)  Indices=1  OutputSizes=1
  Selector2 : Selector  InputPortWidth=128  IndexOptions=Index vector (dialog)  Indices=1  OutputSizes=1
  Selector3 : Selector  InputPortWidth=128  IndexOptions=Index vector (dialog)  Indices=1  OutputSizes=1
  Terminator_3 : Terminator
  Terminator_4 : Terminator
  referenceline info : Outport
  wires:
  [global_path_x] -> MATLAB Function2/2(global_path_x)
  [host_x] -> MATLAB Function6/1(x_set)
  [global_kappa] -> MATLAB Function6/6(frenet_path_kappa)
  [global_yaw] -> MATLAB Function6/5(frenet_path_heading)
  [global_path_y] -> MATLAB Function6/4(frenet_path_y)
  [global_path_x] -> MATLAB Function6/3(frenet_path_x)
  [host_y] -> MATLAB Function6/2(y_set)
  Selector/1 -> [origin_match_point_index], MATLAB Function2/1(host_match_point_index)
  MATLAB Function6/1(match_point_index_set) -> Selector/1
  [global_path_y] -> MATLAB Function2/3(global_path_y)
  Bus Selector/5 -> [host_vy]  "<host_vy>"
  Bus Selector/1 -> [host_x]  "<host_x>"
  Bus Selector/2 -> [host_y]  "<host_y>"
  Bus Selector/3 -> [host_heading_xy]  "<host_heading_xy>"
  Bus Selector/4 -> [host_vx]  "<host_vx>"
  Bus Selector/7 -> [host_speed]  "<host_speed>"
  Bus Selector/6 -> [host_yawrate]  "<host_yawrate>"
  location info/1 -> Bus Selector/1
  [referenceline_x] -> Bus Creator/1  "referenceline_x"
  [referenceline_y] -> Bus Creator/2  "referenceline_y"
  Bus Creator/1 -> referenceline info/1  "referenceline info"
  [referenceline_kappa] -> Bus Creator/4  "referenceline_kappa"
  [referenceline_heading] -> Bus Creator/3  "referenceline_heading"
  [reference_match_point_index] -> Bus Creator/5  "origin_match_point_index"
  [origin_x] -> Bus Creator/6  "origin_x"
  [origin_y] -> Bus Creator/7  "origin_y"
  MATLAB Function6/4(proj_heading_set) -> Terminator_3/1
  MATLAB Function6/5(proj_kappa_set) -> Terminator_4/1
  Constant/1 -> [global_path_x]
  Constant1/1 -> [global_path_y]
  Constant2/1 -> [global_yaw]
  Constant3/1 -> [global_kappa]
  [global_yaw] -> MATLAB Function2/4(global_heading)
  [global_kappa] -> MATLAB Function2/5(global_kappa)
  MATLAB Function2/1(referenceline_x) -> [referenceline_x]
  MATLAB Function2/2(referenceline_y) -> [referenceline_y]
  MATLAB Function2/3(referenceline_heading) -> [referenceline_heading]
  MATLAB Function2/4(referenceline_kappa) -> [referenceline_kappa]
  Selector3/1 -> [origin_y]
  MATLAB Function6/3(proj_y_set) -> Selector3/1
  MATLAB Function6/2(proj_x_set) -> Selector2/1
  Selector2/1 -> [origin_x]
  MATLAB Function2/5(reference_match_point_index) -> [reference_match_point_index]

== system formation_planner_exp_cs/Audi_A8_Sedan_1/Dynamics_UserSpecified/CarSim2PreScanSTATE/Transformation_SprungMassCarSim2PreScan ==
  In1 : Inport
  Demux : Demux  Outputs=3
  Ini z-position VEHICLE wrt GLOBAL axis system [m] : Constant  Value=z0
  Mux : Mux  Inputs=3
  Sum1 : Sum  Inputs=+-
  Out1 : Outport
  wires:
  Mux/1 -> Out1/1
  Ini z-position VEHICLE wrt GLOBAL axis system [m]/1 -> Sum1/2
  Demux/1 -> Mux/1
  Sum1/1 -> Mux/3
  Demux/3 -> Sum1/1
  Demux/2 -> Mux/2
  In1/1 -> Demux/1

== system formation_planner_exp_cs/Audi_A8_Sedan_1/SELF_Demux/compas converter/cart2compas ==
  Angle [deg] : Inport
  Constant : Constant  Value=90
  Constant1 : Constant  Value=360
  Gain : Gain  Gain=1/360
  Gain1 : Gain  Gain=360
  Gain2 : Gain  Gain=-1
  Rounding Function : Rounding
  Sum : Sum  Inputs=|-+
  Sum1 : Sum  Inputs=-+|
  Sum2 : Sum  Inputs=++|
  heading [deg] : Outport
  wires:
  Gain/1 -> Rounding Function/1
  Rounding Function/1 -> Gain1/1
  Gain1/1 -> Sum/1
  Angle [deg]/1 -> Sum1/2
  Sum/1 -> Gain2/1
  Sum1/1 -> Gain/1, Sum/2
  Constant/1 -> Sum1/1
  Gain2/1 -> Sum2/2
  Constant1/1 -> Sum2/1
  Sum2/1 -> heading [deg]/1

== system formation_planner_exp_cs/Audi_A8_Sedan_1/control module1/control main/chassic steering system ==
  LQR_final_angle : Inport
  Constant : Constant  Value=la
  Constant1 : Constant  Value=lb
  Constant17 : Constant  Value=c_factor
  Divide : Product  Inputs=*/
  Gain3 : Gain  Gain=180/pi
  Gain4 : Gain  Gain=360
  MATLAB Function : MATLAB Function  TreatAsAtomicUnit=on
  Saturation : Saturate  UpperLimit=70  LowerLimit=-70
  Saturation1 : Saturate  UpperLimit=1.2217  LowerLimit=-1.2217
  transfer right wheel angle to rack displancement : Lookup_n-D  NumberOfTableDimensions=1  BreakpointsForDimension1=right_wheel_ground  Table=rack_displacement  InternalRulePriority=Speed  RndMeth=Simplest
  lat_steer_sw[deg] : Outport
  wires:
  transfer right wheel angle to rack displancement/1 -> Divide/1
  Constant17/1 -> Divide/2
  Gain4/1 -> lat_steer_sw[deg]/1
  Divide/1 -> Gain4/1
  Saturation/1 -> transfer right wheel angle to rack displancement/1
  Constant/1 -> MATLAB Function/2(la)
  Gain3/1 -> Saturation/1
  Constant1/1 -> MATLAB Function/3(lb)
  LQR_final_angle/1 -> Saturation1/1
  Saturation1/1 -> MATLAB Function/1(u)
  MATLAB Function/1(right_steer) -> Gain3/1

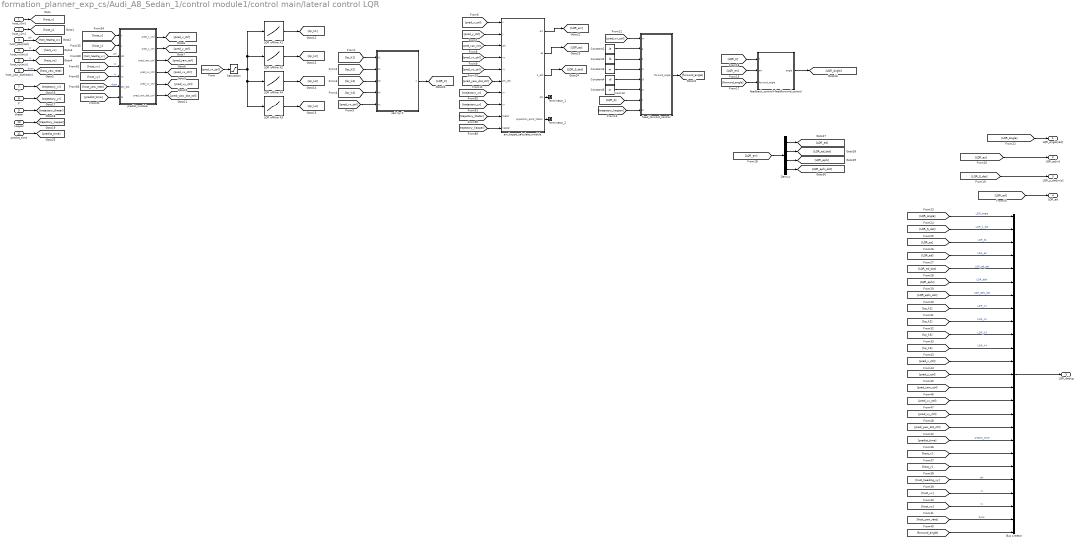
== system formation_planner_exp_cs/Audi_A8_Sedan_1/control module1/control main/lateral control LQR ==
  host_x[m] : Inport
  host_y[m] : Inport  Port=2
  host_yaw[rad] : Inport  Port=3
  host_vx[m/s] : Inport  Port=4
  host_vy[m/s] : Inport  Port=5
  host_yaw_dot[rad/s] : Inport  Port=6
  xr : Inport  Port=7
  yr : Inport  Port=8
  thetar : Inport  Port=9
  kappar : Inport  Port=10
  predict_time : Inport  Port=11
  Bus Creator : BusCreator  Inputs=25
  Constant1 : Constant  Value=la
  Constant2 : Constant  Value=lb
  Constant3 : Constant  Value=m
  Constant4 : Constant  Value=cf
  Constant5 : Constant  Value=cr
  Demux : Demux
  LQR offline K1 : Lookup_n-D  NumberOfTableDimensions=1  BreakpointsForDimension1=vx_break_point  Table=LQR_K1  InternalRulePriority=Speed  RndMeth=Simplest
  LQR offline K2 : Lookup_n-D  NumberOfTableDimensions=1  BreakpointsForDimension1=vx_break_point  Table=LQR_K2  InternalRulePriority=Speed  RndMeth=Simplest
  LQR offline K3 : Lookup_n-D  NumberOfTableDimensions=1  BreakpointsForDimension1=vx_break_point  Table=LQR_K3  InternalRulePriority=Speed  RndMeth=Simplest
  LQR offline K4 : Lookup_n-D  NumberOfTableDimensions=1  BreakpointsForDimension1=vx_break_point  Table=LQR_K4  InternalRulePriority=Speed  RndMeth=Simplest
  Saturation : Saturate  UpperLimit=50  LowerLimit=0
  Terminator_1 : Terminator
  Terminator_2 : Terminator
  calc lqr K : MATLAB Function  TreatAsAtomicUnit=on
  err_kappa_calculate_module : MATLAB Function  TreatAsAtomicUnit=on
  feed_forword_control : MATLAB Function  TreatAsAtomicUnit=on
  feedback_control+feedforword_control : MATLAB Function  TreatAsAtomicUnit=on
  predict_module : MATLAB Function  TreatAsAtomicUnit=on
  LQR_angle[rad] : Outport  VectorParamsAs1DForOutWhenUnconnected=off
  LQR_es[m] : Outport  Port=2  VectorParamsAs1DForOutWhenUnconnected=off
  LQR_s_dot[m/s] : Outport  Port=3  VectorParamsAs1DForOutWhenUnconnected=off
  LQR_ed : Outport  Port=4  VectorParamsAs1DForOutWhenUnconnected=off
  LQR_debug : Outport  Port=5  VectorParamsAs1DForOutWhenUnconnected=off
  wires:
  [host_vy] -> predict_module/5(vy)  "vy"
  [host_x] -> predict_module/1(x)
  [host_yaw_rate] -> predict_module/6(phi_dot)  "dyaw"
  [host_vx] -> predict_module/4(vx)  "vx"
  [host_y] -> predict_module/2(y)
  [host_heading_xy] -> predict_module/3(phi)  "phi"
  [predict_time] -> predict_module/7(ts)
  host_x[m]/1 -> [host_x]
  host_y[m]/1 -> [host_y]
  host_yaw[rad]/1 -> [host_heading_xy]  "phi"
  host_vx[m/s]/1 -> [host_vx]  "vx"
  host_vy[m/s]/1 -> [host_vy]  "vy"
  host_yaw_dot[rad/s]/1 -> [host_yaw_rate]  "dyaw"
  predict_module/1(pred_x_ctrl) -> [pred_x_ctrl]
  predict_module/2(pred_y_ctrl) -> [pred_y_ctrl]
  predict_module/3(pred_yaw_ctrl) -> [pred_yaw_ctrl]
  predict_module/4(pred_vx_ctrl) -> [pred_vx_ctrl]
  predict_module/5(pred_vy_ctrl) -> [pred_vy_ctrl]
  predict_module/6(pred_yaw_dot_ctrl) -> [pred_yaw_dot_ctrl]
  [pred_vx_ctrl] -> Saturation/1
  LQR offline K1/1 -> [lqr_k1]
  LQR offline K2/1 -> [lqr_k2]
  LQR offline K4/1 -> [lqr_k3]
  LQR offline K3/1 -> [lqr_k4]
  [pred_vx_ctrl] -> calc lqr K/5(vx)
  [lqr_k4] -> calc lqr K/4(k4)
  [lqr_k3] -> calc lqr K/3(k3)
  [lqr_k2] -> calc lqr K/2(k2)
  [lqr_k1] -> calc lqr K/1(k1)
  [pred_x_ctrl] -> err_kappa_calculate_module/1(x)
  [pred_y_ctrl] -> err_kappa_calculate_module/2(y)
  [pred_yaw_ctrl] -> err_kappa_calculate_module/3("phi ")
  [pred_vx_ctrl] -> err_kappa_calculate_module/4(vx)
  [pred_vy_ctrl] -> err_kappa_calculate_module/5(vy)
  [pred_yaw_dot_ctrl] -> err_kappa_calculate_module/6(phi_dot)
  xr/1 -> [trajectory_xr]
  yr/1 -> [trajectory_yr]
  thetar/1 -> [trajectory_thetar]
  kappar/1 -> [trajectory_kappar]
  [trajectory_xr] -> err_kappa_calculate_module/7(xr)
  [trajectory_yr] -> err_kappa_calculate_module/8(yr)
  [trajectory_kappar] -> err_kappa_calculate_module/10(kappar)
  [trajectory_thetar] -> err_kappa_calculate_module/9(thetar)
  [pred_vx_ctrl] -> feed_forword_control/1(vx)
  Constant1/1 -> feed_forword_control/2(a)
  Constant2/1 -> feed_forword_control/3(b)
  Constant3/1 -> feed_forword_control/4(m)
  Constant4/1 -> feed_forword_control/5(cf)
  Constant5/1 -> feed_forword_control/6(cr)
  calc lqr K/1(k) -> [LQR_K]
  [LQR_K] -> feed_forword_control/7(k)
  [trajectory_kappar] -> feed_forword_control/8(kr)
  feed_forword_control/1(forword_angle) -> [forword_angle]
  err_kappa_calculate_module/1(err) -> [LQR_err]
  [LQR_err] -> feedback_control+feedforword_control/2(err)
  [LQR_K] -> feedback_control+feedforword_control/1(k)
  [forword_angle] -> feedback_control+feedforword_control/3(forword_angle)
  [LQR_err] -> Demux/1
  err_kappa_calculate_module/2(es) -> [LQR_es]
  err_kappa_calculate_module/3(s_dot) -> [LQR_S_dot]
  [LQR_S_dot] -> LQR_s_dot[m/s]/1
  [LQR_es] -> LQR_es[m]/1
  Saturation/1 -> LQR offline K3/1, LQR offline K4/1, LQR offline K2/1, LQR offline K1/1
  predict_time/1 -> [predict_time]
  Bus Creator/1 -> LQR_debug/1
  feedback_control+feedforword_control/1(angle) -> [LQR_Angle]
  [LQR_Angle] -> LQR_angle[rad]/1
  [LQR_Angle] -> Bus Creator/1  "LQR_angle"
  [LQR_S_dot] -> Bus Creator/2  "LQR_s_dot"
  [LQR_es] -> Bus Creator/3  "LQR_es"
  Demux/1 -> [LQR_ed]
  Demux/2 -> [LQR_ed_dot]
  Demux/3 -> [LQR_ephi]
  Demux/4 -> [LQR_ephi_dot]
  [LQR_ed] -> Bus Creator/4  "LQR_ed"
  [LQR_ed_dot] -> Bus Creator/5  "LQR_ed_dot"
  [LQR_ephi] -> Bus Creator/6  "LQR_ephi"
  [LQR_ephi_dot] -> Bus Creator/7  "LQR_ephi_dot"
  [lqr_k1] -> Bus Creator/8  "LQR_K1"
  [lqr_k2] -> Bus Creator/9  "LQR_K2"
  [lqr_k3] -> Bus Creator/10  "LQR_K3"
  [lqr_k4] -> Bus Creator/11  "LQR_K4"
  [pred_x_ctrl] -> Bus Creator/12
  [pred_y_ctrl] -> Bus Creator/13
  [pred_yaw_ctrl] -> Bus Creator/14
  [pred_vx_ctrl] -> Bus Creator/15
  [pred_vy_ctrl] -> Bus Creator/16
  [pred_yaw_dot_ctrl] -> Bus Creator/17
  [predict_time] -> Bus Creator/18  "predict_time"
  [host_x] -> Bus Creator/19
  [host_y] -> Bus Creator/20
  [host_heading_xy] -> Bus Creator/21  "phi"
  [host_vx] -> Bus Creator/22  "vx"
  [host_vy] -> Bus Creator/23  "vy"
  [host_yaw_rate] -> Bus Creator/24  "dyaw"
  [forword_angle] -> Bus Creator/25
  [LQR_ed] -> LQR_ed/1
  err_kappa_calculate_module/4(phi) -> Terminator_1/1
  err_kappa_calculate_module/5(projection_point_thetar) -> Terminator_2/1
